simulink model "example_Hydraulic_Thermosyphon"  (R2016b)
settings: Solver=ode45  StartTime=0.0  StopTime=3600  RelTol=1e-3  EnableMultiTasking=on
libraries: carnot x7, simulink x1
settings Model: Creator=drhf  LastModifiedBy=drhf
settings DataIOCC: LimitDataPoints=on  SaveFormat=Array  SignalLoggingSaveFormat=ModelDataLogs
settings OptimizationCC: ExpressionDepthLimit=2147483647  LifeSpan=inf
settings DebuggingCC: UnderspecifiedInitializationDetection=Classic  MergeDetectMultiDrivingBlocksExec=none  SolverPrmCheckMsg=warning  FcnCallInpInsideContextMsg=warning  StateNameClashWarn=warning  SFUnexpectedBacktrackingDiag=warning  SFNoUnconditionalDefaultTransitionDiag=warning  SFExecutionAtInitializationDiag=none
settings HardwareCC: ProdBitPerPointer=32  ProdBitPerSizeT=32  ProdBitPerPtrDiffT=32  ProdLargestAtomicFloat=None  ProdIntDivRoundTo=Undefined  ProdEndianess=Unspecified  ProdWordSize=32  ProdHWDeviceType=32-bit Generic
settings ModelReferenceCC: PropagateSignalLabelsOutOfModel=off
settings GRTTargetCC: TargetLangStandard=C89/C90 (ANSI)  GeneratePreprocessorConditionals=Disable all  CombineOutputUpdateFcns=off  GRTInterface=on
settings ConfigComp: CovMetricSettings=dw  CovHtmlReporting=on  CovSaveCumulativeToWorkspaceVar=on  CovSaveSingleToWorkspaceVar=on  CovExternalEMLEnable=off

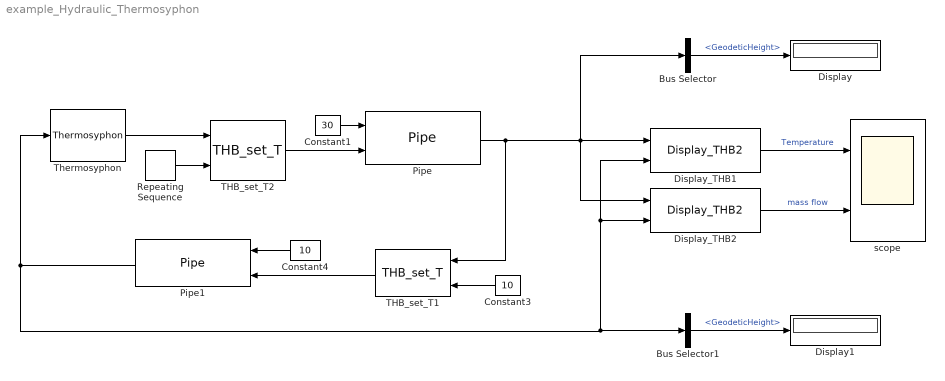
== system example_Hydraulic_Thermosyphon ==
  Bus Selector : BusSelector  OutputSignals=GeodeticHeight
  Bus Selector1 : BusSelector  OutputSignals=GeodeticHeight
  Constant1 : Constant  Value=30
  Constant3 : Constant  Value=10
  Constant4 : Constant  Value=10
  Display : Display
  Display1 : Display
  Display_THB1 : carnot/Outputs/Display_THB2  t=on  m=off  p=off  id=off  mix=off  d=off
  Display_THB2 : carnot/Outputs/Display_THB2  t=off  m=on  p=off  id=off  mix=off  d=off
  Pipe : carnot/Hydraulics/Pipe  dia=0.02  len=10  hgt=5  uloss=100/20/10  cond=0  cwall=1000  t0=10  lin=100/0.2  qua=100/0.2^2  nodes=10
  Pipe1 : carnot/Hydraulics/Pipe  dia=0.02  len=10  hgt=-5  uloss=100/20/10  cond=0  cwall=1000  t0=10  lin=100/0.2  qua=100/0.2^2  nodes=10
  Repeating Sequence : simulink/Sources/Repeating Sequence  rep_seq_t=[0 1 2]*1800  rep_seq_y=[10 50 10]
  THB_set_T1 : carnot/Source/Simple/THB_set_T
  THB_set_T2 : carnot/Source/Simple/THB_set_T
  Thermosyphon : carnot/Hydraulics/Thermosyphon  p0=2e5  dia=0.025  fluid_id=Water  mix=0  mix2=0  mix3=0  t1=5
  scope : Scope  NumInputPorts=2
  wires:
  Display_THB2/1 -> scope/2  "mass flow"
  Pipe1/1 -> Thermosyphon/1, Bus Selector1/1, Display_THB1/2, Display_THB2/2
  Thermosyphon/1 -> THB_set_T2/1
  THB_set_T2/1 -> Pipe/2
  Constant1/1 -> Pipe/1
  Repeating Sequence/1 -> THB_set_T2/2
  THB_set_T1/1 -> Pipe1/2
  Pipe/1 -> THB_set_T1/1, Display_THB1/1, Display_THB2/1, Bus Selector/1
  Constant3/1 -> THB_set_T1/2
  Bus Selector/1 -> Display/1  "<GeodeticHeight>"
  Bus Selector1/1 -> Display1/1  "<GeodeticHeight>"
  Constant4/1 -> Pipe1/1
  Display_THB1/1 -> scope/1  "Temperature"
